simulink model "attitude_control_diagrams_RCAngles"  (Simulink 7.5)
settings: Solver=ode45  StartTime=0.0  StopTime=10.0  RelTol=1e-3
undefined symbols (not defined in the file): Kd, Ki, Kp
settings Model: Creator=tlmolloy  LastModifiedBy=tlmolloy
settings DebuggingCC: StrictBusMsg=Warning

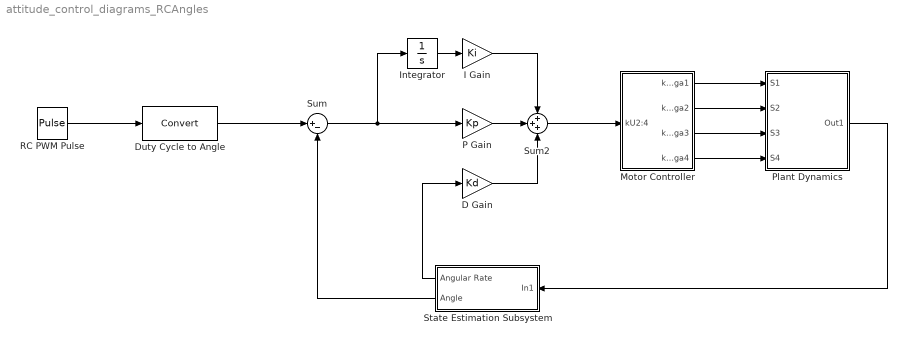
== system attitude_control_diagrams_RCAngles ==
  D Gain : Gain  Gain=Kd  ParameterDataType=fixdt(1, 16)  ParameterScaling=2^0  OutDataType=fixdt(1, 16)  OutScaling=2^0
  Duty Cycle to Angle : DataTypeConversion  OutDataType=fixdt(1, 16)  OutScaling=2^0
  I Gain : Gain  Gain=Ki  ParameterDataType=fixdt(1, 16)  ParameterScaling=2^0  OutDataType=fixdt(1, 16)  OutScaling=2^0
  Integrator : Integrator
  Motor Controller : Subsystem
  P Gain : Gain  Gain=Kp  ParameterDataType=fixdt(1, 16)  ParameterScaling=2^0  OutDataType=fixdt(1, 16)  OutScaling=2^0
  Plant Dynamics : Subsystem
  RC PWM Pulse : DiscretePulseGenerator  PulseType=Time based  Amplitude=1  Period=10  PulseWidth=5  PhaseDelay=0  SampleTime=1
  State Estimation Subsystem : Subsystem
  Sum : Sum  Inputs=|+-  OutDataType=fixdt(1, 16)  OutScaling=2^0
  Sum2 : Sum  Inputs=+++  OutDataType=fixdt(1, 16)  OutScaling=2^0
  wires:
  Sum/1 -> P Gain/1, Integrator/1
  D Gain/1 -> Sum2/3
  P Gain/1 -> Sum2/2
  Integrator/1 -> I Gain/1
  I Gain/1 -> Sum2/1
  Plant Dynamics/1(Out1) -> State Estimation Subsystem/1(In1)
  State Estimation Subsystem/2(Angle) -> Sum/2
  State Estimation Subsystem/1(Angular Rate) -> D Gain/1
  Motor Controller/1(kOmega1) -> Plant Dynamics/1(S1)
  Motor Controller/2(kOmega2) -> Plant Dynamics/2(S2)
  Motor Controller/3(kOmega3) -> Plant Dynamics/3(S3)
  Motor Controller/4(kOmega4) -> Plant Dynamics/4(S4)
  Duty Cycle to Angle/1 -> Sum/1
  Sum2/1 -> Motor Controller/1(kU2:4)
  RC PWM Pulse/1 -> Duty Cycle to Angle/1

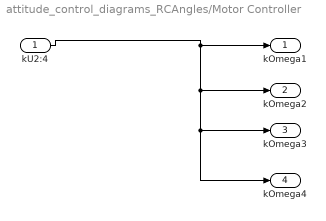
== system attitude_control_diagrams_RCAngles/Motor Controller ==
  kU2:4 : Inport  OutDataType=fixdt(1, 16)  OutScaling=2^0
  kOmega1 : Outport  OutDataType=fixdt(1, 16)  OutScaling=2^0
  kOmega2 : Outport  Port=2  OutDataType=fixdt(1, 16)  OutScaling=2^0
  kOmega3 : Outport  Port=3  OutDataType=fixdt(1, 16)  OutScaling=2^0
  kOmega4 : Outport  Port=4  OutDataType=fixdt(1, 16)  OutScaling=2^0
  wires:
  kU2:4/1 -> kOmega1/1, kOmega2/1, kOmega3/1, kOmega4/1

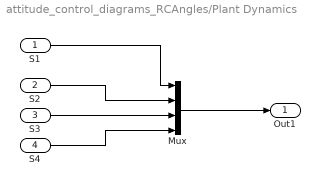
== system attitude_control_diagrams_RCAngles/Plant Dynamics ==
  S1 : Inport  OutDataType=fixdt(1, 16)  OutScaling=2^0
  S2 : Inport  Port=2  OutDataType=fixdt(1, 16)  OutScaling=2^0
  S3 : Inport  Port=3  OutDataType=fixdt(1, 16)  OutScaling=2^0
  S4 : Inport  Port=4  OutDataType=fixdt(1, 16)  OutScaling=2^0
  Mux : Mux
  Out1 : Outport  OutDataType=fixdt(1, 16)  OutScaling=2^0
  wires:
  S2/1 -> Mux/2
  S3/1 -> Mux/3
  S4/1 -> Mux/4
  S1/1 -> Mux/1
  Mux/1 -> Out1/1

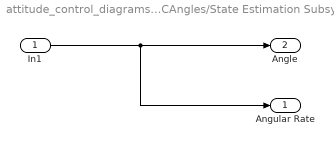
== system attitude_control_diagrams_RCAngles/State Estimation Subsystem ==
  In1 : Inport  OutDataType=fixdt(1, 16)  OutScaling=2^0
  Angular Rate : Outport  OutDataType=fixdt(1, 16)  OutScaling=2^0
  Angle : Outport  Port=2  OutDataType=fixdt(1, 16)  OutScaling=2^0
  wires:
  In1/1 -> Angle/1, Angular Rate/1
